simulink model "HVDCMMCInterconnection"  (R2024b)
settings: Solver=FixedStepDiscrete  StartTime=0.0  StopTime=11  RelTol=1e-3
PreLoadFcn:
  | GFLParameters_400Kv
  | HVDCMMCInterconnectionParam
StartFcn:
  | tic
StopFcn:
  | toc
values from neighbouring files (symbols this model uses):
  C_PM = 1.758e-3    (= 0.001758)    [HVDCMMCInterconnectionParam.m]
  Cfilter = 1/(Larm*wc2)    (= 4.78421193241e-05)    [HVDCMMCInterconnectionParam.m]
  Cg = 50e-9    (= 5e-08)    [HVDCMMCInterconnectionParam.m]
  Fc = Fnom*3.37    (= 168.5)    [HVDCMMCInterconnectionParam.m]
  Fnom = 50    [GFLParameters_400Kv.m]    (also in HVDCMMCInterconnectionParam.m)
  L_cable = 15e-3    (= 0.015)    [HVDCMMCInterconnectionParam.m]
  Larm = Larm_pu*(Zbase/(2*pi*Fnom))    (= 0.0529455974536)    [HVDCMMCInterconnectionParam.m]
  Limits_Qreg = [ 0.25, -0.25 ]    [HVDCMMCInterconnectionParam.m]
  Lxfo = 0.12    [HVDCMMCInterconnectionParam.m]
  Nb_PM = 36    [HVDCMMCInterconnectionParam.m]
  Pnom = 1000e6    (= 1000000000)    [HVDCMMCInterconnectionParam.m]
  Psc = Pnom*20    (= 20000000000)    [HVDCMMCInterconnectionParam.m]    (also in HVDCMMC_RunFaultAnalysis.m = gridSCLArray(k))
  R_cable = 0.5    [HVDCMMCInterconnectionParam.m]
  R_startup = 400    [HVDCMMCInterconnectionParam.m]
  Rarm = Rarm_pu*Zbase    (= 0.1663335)    [HVDCMMCInterconnectionParam.m]
  Rfilter = 1/(Cfilter*w)*30    (= 1996.002)    [HVDCMMCInterconnectionParam.m]
  Rg = 100    [HVDCMMCInterconnectionParam.m]
  Rxfo = 0.003    [HVDCMMCInterconnectionParam.m]
  Slope_Pref = 0.5    [HVDCMMCInterconnectionParam.m]
  Slope_Qref = 0.5    [HVDCMMCInterconnectionParam.m]
  Slope_Vdc_ref = Vnom_dc/5    (= 128000)    [HVDCMMCInterconnectionParam.m]
  Tbrk1_On = 0.1    [HVDCMMCInterconnectionParam.m]
  Tbrk2_On = 1.0    (= 1)    [HVDCMMCInterconnectionParam.m]
  Tdeblock = 1.5    [HVDCMMCInterconnectionParam.m]
  Tfault = 9999    [HVDCMMCInterconnectionParam.m]
  Ton_Converter2 = 4    [HVDCMMCInterconnectionParam.m]
  Ton_PQreg = 4    [HVDCMMCInterconnectionParam.m]
  Ton_VDCreg = 1.5    [HVDCMMCInterconnectionParam.m]
  Ts = Ts_Control    (= 4e-05)    [HVDCMMCInterconnectionParam.m]
  Ts_Power = 20e-6    (= 2e-05)    [HVDCMMCInterconnectionParam.m]
  Vnom_dc = 640e3    (= 640000)    [HVDCMMCInterconnectionParam.m]
  Vnom_prim = 400e3    (= 400000)    [HVDCMMCInterconnectionParam.m]
  Vnom_sec = 333e3    (= 333000)    [HVDCMMCInterconnectionParam.m]
undefined symbols (not defined in the file or in its folder): ConvCtrl, ConvPlt, DiscIntNeverNeededParam, Discrete, ee_sli_rtmsupport, Fault, gcbh, gridInverter, magnitude, Pcc, PlantSim, sps, sps_rtmsupport, spsPLL3phModel, TL, Trf
libraries: powerlib_extras x27, spsSeriesRLCBranchLib x27, simulink x14, eeGeneralControl x11, spsCurrentMeasurementLib x11, spsVoltageMeasurementLib x8, spsBreakerLib x7, eeTransforms x6, spsHalfBridgeMMCLib x6, spsSecondOrderFilterLib x4, spsabctodq0Lib x4, spsThreePhaseVIMeasurementLib x4
(part 3 of 6)

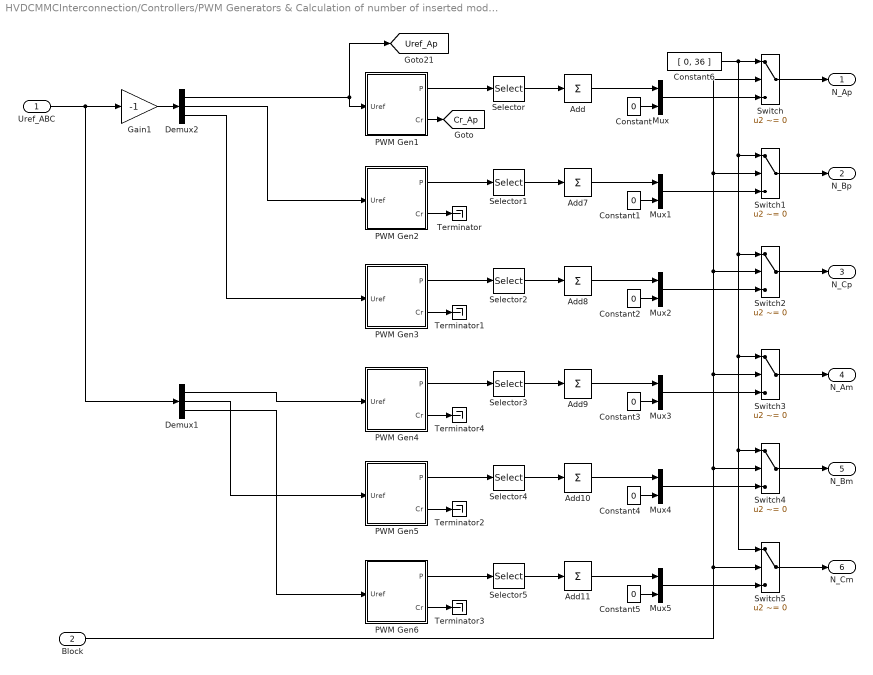
== system HVDCMMCInterconnection/Controllers/PWM Generators & Calculation of number of inserted modules (Nin) and number of blocked module (Nbl) ==
  Uref_ABC : Inport  PortDimensions=3
  Block : Inport  Port=2
  Add{,7..11} (6 alike) : Sum  Inputs=1
  Constant{,1..5} (6 alike) : Constant  Value=0
  Constant6 : Constant  Value=[ 0, 36 ]
  Demux1 : Demux  Outputs=3
  Demux2 : Demux  Outputs=3
  Gain1 : Gain  Gain=-1
  Mux{,1..5} (6 alike) : Mux  Inputs=2
  PWM Gen1 : Subsystem  mask(PWM generator for half-bridge MMC){n=Nb_PM, Fc=Fc, Ts=Ts_Power}
      mask prompts: n "Number of half-bridges"; Fc "Carriers frequency (Hz)"; Ts "Sample time (s)"
      mask init:
      | Tc=1/Fc;
      |         Pc= [ 0:360/n:360-360/n]*pi/180;
      |         Offset=Pc/(2*pi);
      |         Offset_Cr=Pc/(2*pi)*Tc;
      |         p=0;
      |         for m=1:2:2*n
      |             p=p+1;
      |             SelectPulsesPS(m)=p;
      |             SelectPulsesPS(m+1)=p+n;
      |         end
  PWM Gen2 : Subsystem  mask(PWM generator for half-bridge MMC){n=Nb_PM, Fc=Fc, Ts=Ts_Power}
      mask prompts: n "Number of half-bridges"; Fc "Carriers frequency (Hz)"; Ts "Sample time (s)"
      mask init: same as HVDCMMCInterconnection/Controllers/PWM Generators & Calculation of number of inserted modules (Nin) and number of blocked module (Nbl)/PWM Gen1
  PWM Gen3 : Subsystem  mask(PWM generator for half-bridge MMC){n=Nb_PM, Fc=Fc, Ts=Ts_Power}
      mask prompts: n "Number of half-bridges"; Fc "Carriers frequency (Hz)"; Ts "Sample time (s)"
      mask init: same as HVDCMMCInterconnection/Controllers/PWM Generators & Calculation of number of inserted modules (Nin) and number of blocked module (Nbl)/PWM Gen1
  PWM Gen4 : Subsystem  mask(PWM generator for half-bridge MMC){n=Nb_PM, Fc=Fc, Ts=Ts_Power}
      mask prompts: n "Number of half-bridges"; Fc "Carriers frequency (Hz)"; Ts "Sample time (s)"
      mask init: same as HVDCMMCInterconnection/Controllers/PWM Generators & Calculation of number of inserted modules (Nin) and number of blocked module (Nbl)/PWM Gen1
  PWM Gen5 : Subsystem  mask(PWM generator for half-bridge MMC){n=Nb_PM, Fc=Fc, Ts=Ts_Power}
      mask prompts: n "Number of half-bridges"; Fc "Carriers frequency (Hz)"; Ts "Sample time (s)"
      mask init: same as HVDCMMCInterconnection/Controllers/PWM Generators & Calculation of number of inserted modules (Nin) and number of blocked module (Nbl)/PWM Gen1
  PWM Gen6 : Subsystem  mask(PWM generator for half-bridge MMC){n=Nb_PM, Fc=Fc, Ts=Ts_Power}
      mask prompts: n "Number of half-bridges"; Fc "Carriers frequency (Hz)"; Ts "Sample time (s)"
      mask init: same as HVDCMMCInterconnection/Controllers/PWM Generators & Calculation of number of inserted modules (Nin) and number of blocked module (Nbl)/PWM Gen1
  Selector{,1..5} (6 alike) : Selector  InputPortWidth=72  IndexOptions=Index vector (dialog)  Indices=[1:2:71]  OutputSizes=1
  Switch{,1..5} (6 alike) : Switch  Criteria=u2 ~= 0  SaturateOnIntegerOverflow=off  InputSameDT=off
  Terminator{,1..4} (5 alike) : Terminator
  N_Ap : Outport
  N_Bp : Outport  Port=2
  N_Cp : Outport  Port=3
  N_Am : Outport  Port=4
  N_Bm : Outport  Port=5
  N_Cm : Outport  Port=6
  tag scope: Cr_Ap=global, Uref_Ap=global
  wires:
  PWM Gen4/2(Cr) -> Terminator4/1
  PWM Gen5/2(Cr) -> Terminator2/1
  Uref_ABC/1 -> Gain1/1, Demux1/1
  PWM Gen6/2(Cr) -> Terminator3/1
  PWM Gen2/2(Cr) -> Terminator/1
  Demux2/2 -> PWM Gen2/1(Uref)
  Demux2/1 -> PWM Gen1/1(Uref), [Uref_Ap]
  Gain1/1 -> Demux2/1
  PWM Gen1/2(Cr) -> [Cr_Ap]
  PWM Gen3/2(Cr) -> Terminator1/1
  Selector/1 -> Add/1
  Selector1/1 -> Add7/1
  Selector2/1 -> Add8/1
  Selector3/1 -> Add9/1
  Selector4/1 -> Add10/1
  Selector5/1 -> Add11/1
  Constant/1 -> Mux/2
  Add7/1 -> Mux1/1
  Constant1/1 -> Mux1/2
  Constant5/1 -> Mux5/2
  Switch/1 -> N_Ap/1
  Switch3/1 -> N_Am/1
  Mux1/1 -> Switch1/3
  Constant6/1 -> Switch/1, Switch5/1, Switch4/1, Switch3/1, Switch2/1, Switch1/1
  Constant2/1 -> Mux2/2
  Add9/1 -> Mux3/1
  Add8/1 -> Mux2/1
  Mux/1 -> Switch/3
  Switch1/1 -> N_Bp/1
  Constant4/1 -> Mux4/2
  Switch2/1 -> N_Cp/1
  Switch4/1 -> N_Bm/1
  Add/1 -> Mux/1
  Switch5/1 -> N_Cm/1
  Constant3/1 -> Mux3/2
  Add10/1 -> Mux4/1
  Add11/1 -> Mux5/1
  Block/1 -> Switch/2, Switch1/2, Switch2/2, Switch3/2, Switch4/2, Switch5/2
  Mux3/1 -> Switch3/3
  Mux4/1 -> Switch4/3
  Mux5/1 -> Switch5/3
  Mux2/1 -> Switch2/3
  PWM Gen6/1(P) -> Selector5/1
  PWM Gen5/1(P) -> Selector4/1
  PWM Gen4/1(P) -> Selector3/1
  PWM Gen3/1(P) -> Selector2/1
  PWM Gen2/1(P) -> Selector1/1
  PWM Gen1/1(P) -> Selector/1
  Demux2/3 -> PWM Gen3/1(Uref)
  Demux1/1 -> PWM Gen4/1(Uref)
  Demux1/3 -> PWM Gen6/1(Uref)
  Demux1/2 -> PWM Gen5/1(Uref)

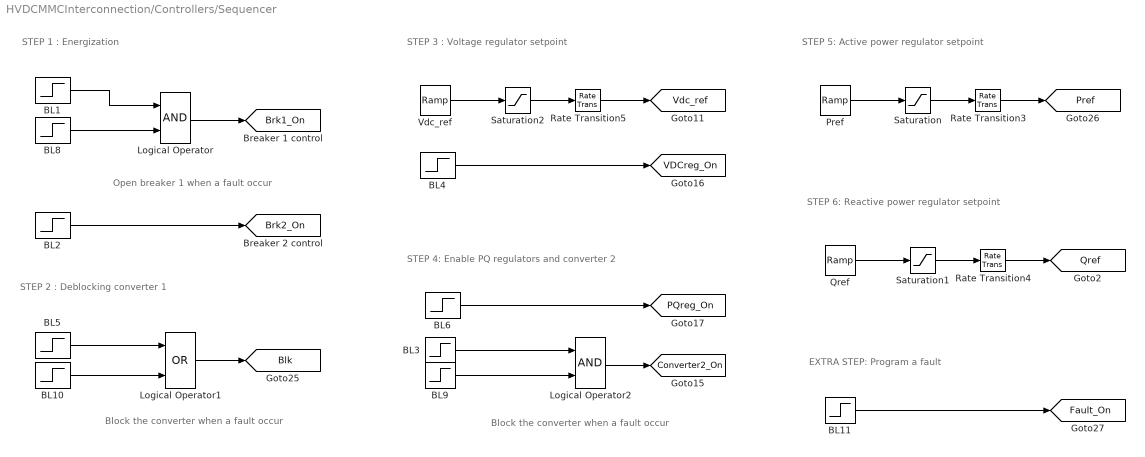
== system HVDCMMCInterconnection/Controllers/Sequencer ==
  note: Open breaker 1 when a fault occur
  note: Block the converter when a fault occur
  note: Block the converter when a fault occur
  note: STEP 6: Reactive power regulator setpoint
  note: STEP 4: Enable PQ regulators and converter 2
  note: STEP 5: Active power regulator setpoint
  note: STEP 3 : Voltage regulator setpoint
  note: STEP 2 : Deblocking converter 1
  note: STEP 1 : Energization
  note: EXTRA STEP: Program a fault
  BL1 : Step  Time=Tbrk1_On  SampleTime=Ts_Power
  BL10 : Step  Time=Tfault+Ts_Power  SampleTime=Ts_Power
  BL11 : Step  Time=Tfault  SampleTime=Ts_Power
  BL2 : Step  Time=Tbrk2_On  SampleTime=Ts_Power
  BL3 : Step  Time=Ton_Converter2  SampleTime=Ts_Power
  BL4 : Step  Time=Ton_VDCreg  SampleTime=Ts
  BL5 : Step  Time=Tdeblock  Before=1  After=0  SampleTime=Ts_Power
  BL6 : Step  Time=Ton_PQreg  SampleTime=Ts
  BL8 : Step  Time=Tfault + 1.95*(1/Fnom)  Before=1  After=0  SampleTime=Ts_Power
  BL9 : Step  Time=Tfault + 2*(1/Fnom)  Before=1  After=0  SampleTime=Ts_Power
  Logical Operator : Logic  AllPortsSameDT=off  OutDataTypeStr=boolean
  Logical Operator1 : Logic  Operator=OR  AllPortsSameDT=off  OutDataTypeStr=float('double')
  Logical Operator2 : Logic  AllPortsSameDT=off  OutDataTypeStr=boolean
  Pref : simulink/Sources/Ramp  slope=Slope_Pref  start=Tramping_Pref  InitialOutput=0
  Qref : simulink/Sources/Ramp  slope=Slope_Qref  start=Tramping_Qref  InitialOutput=0
  Rate Transition3 : RateTransition  OutPortSampleTime=Ts_Control
  Rate Transition4 : RateTransition  OutPortSampleTime=Ts_Control
  Rate Transition5 : RateTransition  OutPortSampleTime=Ts_Control
  Saturation : Saturate  UpperLimit=1  LowerLimit=-1
  Saturation1 : Saturate  UpperLimit=Limits_Qreg(1)  LowerLimit=Limits_Qreg(2)
  Saturation2 : Saturate  UpperLimit=Vnom_dc  LowerLimit=eps
  "Vdc_ref " : simulink/Sources/Ramp  slope=Slope_Vdc_ref  start=Tramping_Vdc_ref  InitialOutput=Vnom_sec*1.37
  tag scope: Blk=global, Brk1_On=global, Brk2_On=global, Converter2_On=global, Fault_On=global, PQreg_On=global, Pref=global, Qref=global, VDCreg_On=global, Vdc_ref=global
  wires:
  Saturation2/1 -> Rate Transition5/1
  Saturation1/1 -> Rate Transition4/1
  Pref/1 -> Saturation/1
  Qref/1 -> Saturation1/1
  Saturation/1 -> Rate Transition3/1
  Rate Transition3/1 -> [Pref]
  Rate Transition4/1 -> [Qref]
  Rate Transition5/1 -> [Vdc_ref]
  BL4/1 -> [VDCreg_On]
  BL6/1 -> [PQreg_On]
  "Vdc_ref "/1 -> Saturation2/1
  BL2/1 -> [Brk2_On]
  BL8/1 -> Logical Operator/2
  Logical Operator/1 -> [Brk1_On]
  BL1/1 -> Logical Operator/1
  BL9/1 -> Logical Operator2/2
  BL3/1 -> Logical Operator2/1
  Logical Operator2/1 -> [Converter2_On]
  Logical Operator1/1 -> [Blk]
  BL5/1 -> Logical Operator1/1
  BL10/1 -> Logical Operator1/2
  BL11/1 -> [Fault_On]

== system HVDCMMCInterconnection/Record Simulation Data/FaultTrigger ==
  mZ1L_Est : Inport
  V1_Local : Inport  Port=2
  I1_Local : Inport  Port=3
  V1_Remote : Inport  Port=4
  I1_Remote : Inport  Port=5
  IdRef : Inport  Port=6
  IqRef : Inport  Port=7
  IdMeas : Inport  Port=8
  IqMeas : Inport  Port=9
  Is : Inport  Port=10
  Vmd : Inport  Port=11
  Vmq : Inport  Port=12
  delVd : Inport  Port=13
  delVq : Inport  Port=14
  Enable : EnablePort
  To Workspace : ToWorkspace  VariableName=mZ1L_Est  SaveFormat=Timeseries  SampleTime=-1
  To Workspace1 : ToWorkspace  VariableName=V1_Local  SaveFormat=Timeseries  SampleTime=-1
  To Workspace10 : ToWorkspace  VariableName=Vmd  SaveFormat=Timeseries  SampleTime=-1
  To Workspace11 : ToWorkspace  VariableName=Vmq  SaveFormat=Timeseries  SampleTime=-1
  To Workspace12 : ToWorkspace  VariableName=delVd  SaveFormat=Timeseries  SampleTime=-1
  To Workspace13 : ToWorkspace  VariableName=delVq  SaveFormat=Timeseries  SampleTime=-1
  To Workspace2 : ToWorkspace  VariableName=I1_Local  SaveFormat=Timeseries  SampleTime=-1
  To Workspace3 : ToWorkspace  VariableName=V1_Remote  SaveFormat=Timeseries  SampleTime=-1
  To Workspace4 : ToWorkspace  VariableName=I1_Remote  SaveFormat=Timeseries  SampleTime=-1
  To Workspace5 : ToWorkspace  VariableName=IdRef  SaveFormat=Timeseries  SampleTime=-1
  To Workspace6 : ToWorkspace  VariableName=IqRef  SaveFormat=Timeseries  SampleTime=-1
  To Workspace7 : ToWorkspace  VariableName=IdMeas  SaveFormat=Timeseries  SampleTime=-1
  To Workspace8 : ToWorkspace  VariableName=IqMeas  SaveFormat=Timeseries  SampleTime=-1
  To Workspace9 : ToWorkspace  VariableName=Is  SaveFormat=Timeseries  SampleTime=-1
  wires:
  mZ1L_Est/1 -> To Workspace/1
  V1_Local/1 -> To Workspace1/1
  I1_Local/1 -> To Workspace2/1
  V1_Remote/1 -> To Workspace3/1
  I1_Remote/1 -> To Workspace4/1
  IdRef/1 -> To Workspace5/1
  IqRef/1 -> To Workspace6/1
  IdMeas/1 -> To Workspace7/1
  IqMeas/1 -> To Workspace8/1
  Is/1 -> To Workspace9/1
  Vmd/1 -> To Workspace10/1
  Vmq/1 -> To Workspace11/1
  delVd/1 -> To Workspace12/1
  delVq/1 -> To Workspace13/1

== system HVDCMMCInterconnection/BusCalculations/Measurement Unit (Phasor Computation)/Discrete Fourier(A) ==
  note: Discrete Fourier
  note: Pierre Giroux, Gilbert Sybille
      | Power System Simulation Laboratory
      | IREQ, Hydro-Quebc
  In : Inport
  Demux : Demux  Outputs=2
      settings: DisplayOption=none
  Discrete Mean value1 : powerlib_extras/Discrete Measurements/Discrete  Mean value  Freq=Freq  Vinit=Real_Init  Ts=Ts
  Discrete Mean value2 : powerlib_extras/Discrete Measurements/Discrete  Mean value  Freq=Freq  Vinit=Imag_Init  Ts=Ts
  Gain : Gain  Gain=2*pi*n*Freq  SaturateOnIntegerOverflow=on  OutDataTypeStr=Inherit: Same as input  ParamDataTypeStr=Inherit: Same as input
  Gain1 : Gain  Gain=k  SaturateOnIntegerOverflow=on  OutDataTypeStr=Inherit: Same as input  ParamDataTypeStr=Inherit: Same as input
  Mux : Mux  Inputs=2
  Product : Product  InputSameDT=on  SaturateOnIntegerOverflow=on  OutDataTypeStr=Inherit: Same as first input
  Real-Imag to Complex : RealImagToComplex
  Trigonometric Function : Trigonometry
  Trigonometric Function1 : Trigonometry  Operator=cos
  t : DigitalClock  SampleTime=Ts
  Fund : Outport
  wires:
  Real-Imag to Complex/1 -> Fund/1
  Discrete Mean value2/1 -> Real-Imag to Complex/2  "Imag"
  Discrete Mean value1/1 -> Real-Imag to Complex/1  "Real"
  t/1 -> Gain/1
  Gain/1 -> Trigonometric Function/1, Trigonometric Function1/1
  Trigonometric Function/1 -> Mux/1
  Trigonometric Function1/1 -> Mux/2
  Mux/1 -> Gain1/1
  In/1 -> Product/1
  Gain1/1 -> Product/2
  Product/1 -> Demux/1
  Demux/1 -> Discrete Mean value1/1
  Demux/2 -> Discrete Mean value2/1

== system HVDCMMCInterconnection/BusCalculations/Measurement Unit (Phasor Computation)/Discrete Fourier(A)  ==
  note: Pierre Giroux, Gilbert Sybille
      | Power System Simulation Laboratory
      | IREQ, Hydro-Quebc
  note: Discrete Fourier
  In : Inport
  Demux : Demux  Outputs=2
      settings: DisplayOption=none
  Discrete Mean value1 : powerlib_extras/Discrete Measurements/Discrete  Mean value  Freq=Freq  Vinit=Real_Init  Ts=Ts
  Discrete Mean value2 : powerlib_extras/Discrete Measurements/Discrete  Mean value  Freq=Freq  Vinit=Imag_Init  Ts=Ts
  Gain : Gain  Gain=2*pi*n*Freq  SaturateOnIntegerOverflow=on  OutDataTypeStr=Inherit: Same as input  ParamDataTypeStr=Inherit: Same as input
  Gain1 : Gain  Gain=k  SaturateOnIntegerOverflow=on  OutDataTypeStr=Inherit: Same as input  ParamDataTypeStr=Inherit: Same as input
  Mux : Mux  Inputs=2
  Product : Product  InputSameDT=on  SaturateOnIntegerOverflow=on  OutDataTypeStr=Inherit: Same as first input
  Real-Imag to Complex : RealImagToComplex
  Trigonometric Function : Trigonometry
  Trigonometric Function1 : Trigonometry  Operator=cos
  t : DigitalClock  SampleTime=Ts
  Fund : Outport
  wires:
  Demux/2 -> Discrete Mean value2/1
  Demux/1 -> Discrete Mean value1/1
  Product/1 -> Demux/1
  Gain1/1 -> Product/2
  In/1 -> Product/1
  Mux/1 -> Gain1/1
  Trigonometric Function1/1 -> Mux/2
  Trigonometric Function/1 -> Mux/1
  Gain/1 -> Trigonometric Function1/1, Trigonometric Function/1
  t/1 -> Gain/1
  Discrete Mean value1/1 -> Real-Imag to Complex/1  "Real"
  Discrete Mean value2/1 -> Real-Imag to Complex/2  "Imag"
  Real-Imag to Complex/1 -> Fund/1

== system HVDCMMCInterconnection/BusCalculations/Measurement Unit (Phasor Computation)/Discrete Fourier(B) ==
  note: Pierre Giroux, Gilbert Sybille
      | Power System Simulation Laboratory
      | IREQ, Hydro-Quebc
  note: Discrete Fourier
  In : Inport
  Demux : Demux  Outputs=2
      settings: DisplayOption=none
  Discrete Mean value1 : powerlib_extras/Discrete Measurements/Discrete  Mean value  Freq=Freq  Vinit=Real_Init  Ts=Ts
  Discrete Mean value2 : powerlib_extras/Discrete Measurements/Discrete  Mean value  Freq=Freq  Vinit=Imag_Init  Ts=Ts
  Gain : Gain  Gain=2*pi*n*Freq  SaturateOnIntegerOverflow=on  OutDataTypeStr=Inherit: Same as input  ParamDataTypeStr=Inherit: Same as input
  Gain1 : Gain  Gain=k  SaturateOnIntegerOverflow=on  OutDataTypeStr=Inherit: Same as input  ParamDataTypeStr=Inherit: Same as input
  Mux : Mux  Inputs=2
  Product : Product  InputSameDT=on  SaturateOnIntegerOverflow=on  OutDataTypeStr=Inherit: Same as first input
  Real-Imag to Complex : RealImagToComplex
  Trigonometric Function : Trigonometry
  Trigonometric Function1 : Trigonometry  Operator=cos
  t : DigitalClock  SampleTime=Ts
  Fund : Outport
  wires:
  Demux/2 -> Discrete Mean value2/1
  Demux/1 -> Discrete Mean value1/1
  Product/1 -> Demux/1
  Gain1/1 -> Product/2
  In/1 -> Product/1
  Mux/1 -> Gain1/1
  Trigonometric Function1/1 -> Mux/2
  Trigonometric Function/1 -> Mux/1
  Gain/1 -> Trigonometric Function1/1, Trigonometric Function/1
  t/1 -> Gain/1
  Discrete Mean value1/1 -> Real-Imag to Complex/1  "Real"
  Discrete Mean value2/1 -> Real-Imag to Complex/2  "Imag"
  Real-Imag to Complex/1 -> Fund/1

== system HVDCMMCInterconnection/BusCalculations/Measurement Unit (Phasor Computation)/Discrete Fourier(B)  ==
  note: Discrete Fourier
  note: Pierre Giroux, Gilbert Sybille
      | Power System Simulation Laboratory
      | IREQ, Hydro-Quebc
  In : Inport
  Demux : Demux  Outputs=2
      settings: DisplayOption=none
  Discrete Mean value1 : powerlib_extras/Discrete Measurements/Discrete  Mean value  Freq=Freq  Vinit=Real_Init  Ts=Ts
  Discrete Mean value2 : powerlib_extras/Discrete Measurements/Discrete  Mean value  Freq=Freq  Vinit=Imag_Init  Ts=Ts
  Gain : Gain  Gain=2*pi*n*Freq  SaturateOnIntegerOverflow=on  OutDataTypeStr=Inherit: Same as input  ParamDataTypeStr=Inherit: Same as input
  Gain1 : Gain  Gain=k  SaturateOnIntegerOverflow=on  OutDataTypeStr=Inherit: Same as input  ParamDataTypeStr=Inherit: Same as input
  Mux : Mux  Inputs=2
  Product : Product  InputSameDT=on  SaturateOnIntegerOverflow=on  OutDataTypeStr=Inherit: Same as first input
  Real-Imag to Complex : RealImagToComplex
  Trigonometric Function : Trigonometry
  Trigonometric Function1 : Trigonometry  Operator=cos
  t : DigitalClock  SampleTime=Ts
  Fund : Outport
  wires:
  Real-Imag to Complex/1 -> Fund/1
  Discrete Mean value2/1 -> Real-Imag to Complex/2  "Imag"
  Discrete Mean value1/1 -> Real-Imag to Complex/1  "Real"
  t/1 -> Gain/1
  Gain/1 -> Trigonometric Function/1, Trigonometric Function1/1
  Trigonometric Function/1 -> Mux/1
  Trigonometric Function1/1 -> Mux/2
  Mux/1 -> Gain1/1
  In/1 -> Product/1
  Gain1/1 -> Product/2
  Product/1 -> Demux/1
  Demux/1 -> Discrete Mean value1/1
  Demux/2 -> Discrete Mean value2/1

== system HVDCMMCInterconnection/BusCalculations/Measurement Unit (Phasor Computation)/Discrete Fourier(C) ==
  note: Discrete Fourier
  note: Pierre Giroux, Gilbert Sybille
      | Power System Simulation Laboratory
      | IREQ, Hydro-Quebc
  In : Inport
  Demux : Demux  Outputs=2
      settings: DisplayOption=none
  Discrete Mean value1 : powerlib_extras/Discrete Measurements/Discrete  Mean value  Freq=Freq  Vinit=Real_Init  Ts=Ts
  Discrete Mean value2 : powerlib_extras/Discrete Measurements/Discrete  Mean value  Freq=Freq  Vinit=Imag_Init  Ts=Ts
  Gain : Gain  Gain=2*pi*n*Freq  SaturateOnIntegerOverflow=on  OutDataTypeStr=Inherit: Same as input  ParamDataTypeStr=Inherit: Same as input
  Gain1 : Gain  Gain=k  SaturateOnIntegerOverflow=on  OutDataTypeStr=Inherit: Same as input  ParamDataTypeStr=Inherit: Same as input
  Mux : Mux  Inputs=2
  Product : Product  InputSameDT=on  SaturateOnIntegerOverflow=on  OutDataTypeStr=Inherit: Same as first input
  Real-Imag to Complex : RealImagToComplex
  Trigonometric Function : Trigonometry
  Trigonometric Function1 : Trigonometry  Operator=cos
  t : DigitalClock  SampleTime=Ts
  Fund : Outport
  wires:
  Real-Imag to Complex/1 -> Fund/1
  Discrete Mean value2/1 -> Real-Imag to Complex/2  "Imag"
  Discrete Mean value1/1 -> Real-Imag to Complex/1  "Real"
  t/1 -> Gain/1
  Gain/1 -> Trigonometric Function/1, Trigonometric Function1/1
  Trigonometric Function/1 -> Mux/1
  Trigonometric Function1/1 -> Mux/2
  Mux/1 -> Gain1/1
  In/1 -> Product/1
  Gain1/1 -> Product/2
  Product/1 -> Demux/1
  Demux/1 -> Discrete Mean value1/1
  Demux/2 -> Discrete Mean value2/1

== system HVDCMMCInterconnection/BusCalculations/Measurement Unit (Phasor Computation)/Discrete Fourier(C)  ==
  note: Pierre Giroux, Gilbert Sybille
      | Power System Simulation Laboratory
      | IREQ, Hydro-Quebc
  note: Discrete Fourier
  In : Inport
  Demux : Demux  Outputs=2
      settings: DisplayOption=none
  Discrete Mean value1 : powerlib_extras/Discrete Measurements/Discrete  Mean value  Freq=Freq  Vinit=Real_Init  Ts=Ts
  Discrete Mean value2 : powerlib_extras/Discrete Measurements/Discrete  Mean value  Freq=Freq  Vinit=Imag_Init  Ts=Ts
  Gain : Gain  Gain=2*pi*n*Freq  SaturateOnIntegerOverflow=on  OutDataTypeStr=Inherit: Same as input  ParamDataTypeStr=Inherit: Same as input
  Gain1 : Gain  Gain=k  SaturateOnIntegerOverflow=on  OutDataTypeStr=Inherit: Same as input  ParamDataTypeStr=Inherit: Same as input
  Mux : Mux  Inputs=2
  Product : Product  InputSameDT=on  SaturateOnIntegerOverflow=on  OutDataTypeStr=Inherit: Same as first input
  Real-Imag to Complex : RealImagToComplex
  Trigonometric Function : Trigonometry
  Trigonometric Function1 : Trigonometry  Operator=cos
  t : DigitalClock  SampleTime=Ts
  Fund : Outport
  wires:
  Demux/2 -> Discrete Mean value2/1
  Demux/1 -> Discrete Mean value1/1
  Product/1 -> Demux/1
  Gain1/1 -> Product/2
  In/1 -> Product/1
  Mux/1 -> Gain1/1
  Trigonometric Function1/1 -> Mux/2
  Trigonometric Function/1 -> Mux/1
  Gain/1 -> Trigonometric Function1/1, Trigonometric Function/1
  t/1 -> Gain/1
  Discrete Mean value1/1 -> Real-Imag to Complex/1  "Real"
  Discrete Mean value2/1 -> Real-Imag to Complex/2  "Imag"
  Real-Imag to Complex/1 -> Fund/1

== system HVDCMMCInterconnection/BusCalculations1/Measurement Unit (Phasor Computation)/Discrete Fourier(A) ==
  note: Pierre Giroux, Gilbert Sybille
      | Power System Simulation Laboratory
      | IREQ, Hydro-Quebc
  note: Discrete Fourier
  In : Inport
  Demux : Demux  Outputs=2
      settings: DisplayOption=none
  Discrete Mean value1 : powerlib_extras/Discrete Measurements/Discrete  Mean value  Freq=Freq  Vinit=Real_Init  Ts=Ts
  Discrete Mean value2 : powerlib_extras/Discrete Measurements/Discrete  Mean value  Freq=Freq  Vinit=Imag_Init  Ts=Ts
  Gain : Gain  Gain=2*pi*n*Freq  SaturateOnIntegerOverflow=on  OutDataTypeStr=Inherit: Same as input  ParamDataTypeStr=Inherit: Same as input
  Gain1 : Gain  Gain=k  SaturateOnIntegerOverflow=on  OutDataTypeStr=Inherit: Same as input  ParamDataTypeStr=Inherit: Same as input
  Mux : Mux  Inputs=2
  Product : Product  InputSameDT=on  SaturateOnIntegerOverflow=on  OutDataTypeStr=Inherit: Same as first input
  Real-Imag to Complex : RealImagToComplex
  Trigonometric Function : Trigonometry
  Trigonometric Function1 : Trigonometry  Operator=cos
  t : DigitalClock  SampleTime=Ts
  Fund : Outport
  wires:
  Demux/2 -> Discrete Mean value2/1
  Demux/1 -> Discrete Mean value1/1
  Product/1 -> Demux/1
  Gain1/1 -> Product/2
  In/1 -> Product/1
  Mux/1 -> Gain1/1
  Trigonometric Function1/1 -> Mux/2
  Trigonometric Function/1 -> Mux/1
  Gain/1 -> Trigonometric Function1/1, Trigonometric Function/1
  t/1 -> Gain/1
  Discrete Mean value1/1 -> Real-Imag to Complex/1  "Real"
  Discrete Mean value2/1 -> Real-Imag to Complex/2  "Imag"
  Real-Imag to Complex/1 -> Fund/1

== system HVDCMMCInterconnection/BusCalculations1/Measurement Unit (Phasor Computation)/Discrete Fourier(A)  ==
  note: Discrete Fourier
  note: Pierre Giroux, Gilbert Sybille
      | Power System Simulation Laboratory
      | IREQ, Hydro-Quebc
  In : Inport
  Demux : Demux  Outputs=2
      settings: DisplayOption=none
  Discrete Mean value1 : powerlib_extras/Discrete Measurements/Discrete  Mean value  Freq=Freq  Vinit=Real_Init  Ts=Ts
  Discrete Mean value2 : powerlib_extras/Discrete Measurements/Discrete  Mean value  Freq=Freq  Vinit=Imag_Init  Ts=Ts
  Gain : Gain  Gain=2*pi*n*Freq  SaturateOnIntegerOverflow=on  OutDataTypeStr=Inherit: Same as input  ParamDataTypeStr=Inherit: Same as input
  Gain1 : Gain  Gain=k  SaturateOnIntegerOverflow=on  OutDataTypeStr=Inherit: Same as input  ParamDataTypeStr=Inherit: Same as input
  Mux : Mux  Inputs=2
  Product : Product  InputSameDT=on  SaturateOnIntegerOverflow=on  OutDataTypeStr=Inherit: Same as first input
  Real-Imag to Complex : RealImagToComplex
  Trigonometric Function : Trigonometry
  Trigonometric Function1 : Trigonometry  Operator=cos
  t : DigitalClock  SampleTime=Ts
  Fund : Outport
  wires:
  Real-Imag to Complex/1 -> Fund/1
  Discrete Mean value2/1 -> Real-Imag to Complex/2  "Imag"
  Discrete Mean value1/1 -> Real-Imag to Complex/1  "Real"
  t/1 -> Gain/1
  Gain/1 -> Trigonometric Function/1, Trigonometric Function1/1
  Trigonometric Function/1 -> Mux/1
  Trigonometric Function1/1 -> Mux/2
  Mux/1 -> Gain1/1
  In/1 -> Product/1
  Gain1/1 -> Product/2
  Product/1 -> Demux/1
  Demux/1 -> Discrete Mean value1/1
  Demux/2 -> Discrete Mean value2/1

== system HVDCMMCInterconnection/BusCalculations1/Measurement Unit (Phasor Computation)/Discrete Fourier(B) ==
  note: Discrete Fourier
  note: Pierre Giroux, Gilbert Sybille
      | Power System Simulation Laboratory
      | IREQ, Hydro-Quebc
  In : Inport
  Demux : Demux  Outputs=2
      settings: DisplayOption=none
  Discrete Mean value1 : powerlib_extras/Discrete Measurements/Discrete  Mean value  Freq=Freq  Vinit=Real_Init  Ts=Ts
  Discrete Mean value2 : powerlib_extras/Discrete Measurements/Discrete  Mean value  Freq=Freq  Vinit=Imag_Init  Ts=Ts
  Gain : Gain  Gain=2*pi*n*Freq  SaturateOnIntegerOverflow=on  OutDataTypeStr=Inherit: Same as input  ParamDataTypeStr=Inherit: Same as input
  Gain1 : Gain  Gain=k  SaturateOnIntegerOverflow=on  OutDataTypeStr=Inherit: Same as input  ParamDataTypeStr=Inherit: Same as input
  Mux : Mux  Inputs=2
  Product : Product  InputSameDT=on  SaturateOnIntegerOverflow=on  OutDataTypeStr=Inherit: Same as first input
  Real-Imag to Complex : RealImagToComplex
  Trigonometric Function : Trigonometry
  Trigonometric Function1 : Trigonometry  Operator=cos
  t : DigitalClock  SampleTime=Ts
  Fund : Outport
  wires:
  Real-Imag to Complex/1 -> Fund/1
  Discrete Mean value2/1 -> Real-Imag to Complex/2  "Imag"
  Discrete Mean value1/1 -> Real-Imag to Complex/1  "Real"
  t/1 -> Gain/1
  Gain/1 -> Trigonometric Function/1, Trigonometric Function1/1
  Trigonometric Function/1 -> Mux/1
  Trigonometric Function1/1 -> Mux/2
  Mux/1 -> Gain1/1
  In/1 -> Product/1
  Gain1/1 -> Product/2
  Product/1 -> Demux/1
  Demux/1 -> Discrete Mean value1/1
  Demux/2 -> Discrete Mean value2/1

== system HVDCMMCInterconnection/BusCalculations1/Measurement Unit (Phasor Computation)/Discrete Fourier(B)  ==
  note: Pierre Giroux, Gilbert Sybille
      | Power System Simulation Laboratory
      | IREQ, Hydro-Quebc
  note: Discrete Fourier
  In : Inport
  Demux : Demux  Outputs=2
      settings: DisplayOption=none
  Discrete Mean value1 : powerlib_extras/Discrete Measurements/Discrete  Mean value  Freq=Freq  Vinit=Real_Init  Ts=Ts
  Discrete Mean value2 : powerlib_extras/Discrete Measurements/Discrete  Mean value  Freq=Freq  Vinit=Imag_Init  Ts=Ts
  Gain : Gain  Gain=2*pi*n*Freq  SaturateOnIntegerOverflow=on  OutDataTypeStr=Inherit: Same as input  ParamDataTypeStr=Inherit: Same as input
  Gain1 : Gain  Gain=k  SaturateOnIntegerOverflow=on  OutDataTypeStr=Inherit: Same as input  ParamDataTypeStr=Inherit: Same as input
  Mux : Mux  Inputs=2
  Product : Product  InputSameDT=on  SaturateOnIntegerOverflow=on  OutDataTypeStr=Inherit: Same as first input
  Real-Imag to Complex : RealImagToComplex
  Trigonometric Function : Trigonometry
  Trigonometric Function1 : Trigonometry  Operator=cos
  t : DigitalClock  SampleTime=Ts
  Fund : Outport
  wires:
  Demux/2 -> Discrete Mean value2/1
  Demux/1 -> Discrete Mean value1/1
  Product/1 -> Demux/1
  Gain1/1 -> Product/2
  In/1 -> Product/1
  Mux/1 -> Gain1/1
  Trigonometric Function1/1 -> Mux/2
  Trigonometric Function/1 -> Mux/1
  Gain/1 -> Trigonometric Function1/1, Trigonometric Function/1
  t/1 -> Gain/1
  Discrete Mean value1/1 -> Real-Imag to Complex/1  "Real"
  Discrete Mean value2/1 -> Real-Imag to Complex/2  "Imag"
  Real-Imag to Complex/1 -> Fund/1

== system HVDCMMCInterconnection/BusCalculations1/Measurement Unit (Phasor Computation)/Discrete Fourier(C) ==
  note: Pierre Giroux, Gilbert Sybille
      | Power System Simulation Laboratory
      | IREQ, Hydro-Quebc
  note: Discrete Fourier
  In : Inport
  Demux : Demux  Outputs=2
      settings: DisplayOption=none
  Discrete Mean value1 : powerlib_extras/Discrete Measurements/Discrete  Mean value  Freq=Freq  Vinit=Real_Init  Ts=Ts
  Discrete Mean value2 : powerlib_extras/Discrete Measurements/Discrete  Mean value  Freq=Freq  Vinit=Imag_Init  Ts=Ts
  Gain : Gain  Gain=2*pi*n*Freq  SaturateOnIntegerOverflow=on  OutDataTypeStr=Inherit: Same as input  ParamDataTypeStr=Inherit: Same as input
  Gain1 : Gain  Gain=k  SaturateOnIntegerOverflow=on  OutDataTypeStr=Inherit: Same as input  ParamDataTypeStr=Inherit: Same as input
  Mux : Mux  Inputs=2
  Product : Product  InputSameDT=on  SaturateOnIntegerOverflow=on  OutDataTypeStr=Inherit: Same as first input
  Real-Imag to Complex : RealImagToComplex
  Trigonometric Function : Trigonometry
  Trigonometric Function1 : Trigonometry  Operator=cos
  t : DigitalClock  SampleTime=Ts
  Fund : Outport
  wires:
  Demux/2 -> Discrete Mean value2/1
  Demux/1 -> Discrete Mean value1/1
  Product/1 -> Demux/1
  Gain1/1 -> Product/2
  In/1 -> Product/1
  Mux/1 -> Gain1/1
  Trigonometric Function1/1 -> Mux/2
  Trigonometric Function/1 -> Mux/1
  Gain/1 -> Trigonometric Function1/1, Trigonometric Function/1
  t/1 -> Gain/1
  Discrete Mean value1/1 -> Real-Imag to Complex/1  "Real"
  Discrete Mean value2/1 -> Real-Imag to Complex/2  "Imag"
  Real-Imag to Complex/1 -> Fund/1

== system HVDCMMCInterconnection/BusCalculations1/Measurement Unit (Phasor Computation)/Discrete Fourier(C)  ==
  note: Discrete Fourier
  note: Pierre Giroux, Gilbert Sybille
      | Power System Simulation Laboratory
      | IREQ, Hydro-Quebc
  In : Inport
  Demux : Demux  Outputs=2
      settings: DisplayOption=none
  Discrete Mean value1 : powerlib_extras/Discrete Measurements/Discrete  Mean value  Freq=Freq  Vinit=Real_Init  Ts=Ts
  Discrete Mean value2 : powerlib_extras/Discrete Measurements/Discrete  Mean value  Freq=Freq  Vinit=Imag_Init  Ts=Ts
  Gain : Gain  Gain=2*pi*n*Freq  SaturateOnIntegerOverflow=on  OutDataTypeStr=Inherit: Same as input  ParamDataTypeStr=Inherit: Same as input
  Gain1 : Gain  Gain=k  SaturateOnIntegerOverflow=on  OutDataTypeStr=Inherit: Same as input  ParamDataTypeStr=Inherit: Same as input
  Mux : Mux  Inputs=2
  Product : Product  InputSameDT=on  SaturateOnIntegerOverflow=on  OutDataTypeStr=Inherit: Same as first input
  Real-Imag to Complex : RealImagToComplex
  Trigonometric Function : Trigonometry
  Trigonometric Function1 : Trigonometry  Operator=cos
  t : DigitalClock  SampleTime=Ts
  Fund : Outport
  wires:
  Real-Imag to Complex/1 -> Fund/1
  Discrete Mean value2/1 -> Real-Imag to Complex/2  "Imag"
  Discrete Mean value1/1 -> Real-Imag to Complex/1  "Real"
  t/1 -> Gain/1
  Gain/1 -> Trigonometric Function/1, Trigonometric Function1/1
  Trigonometric Function/1 -> Mux/1
  Trigonometric Function1/1 -> Mux/2
  Mux/1 -> Gain1/1
  In/1 -> Product/1
  Gain1/1 -> Product/2
  Product/1 -> Demux/1
  Demux/1 -> Discrete Mean value1/1
  Demux/2 -> Discrete Mean value2/1

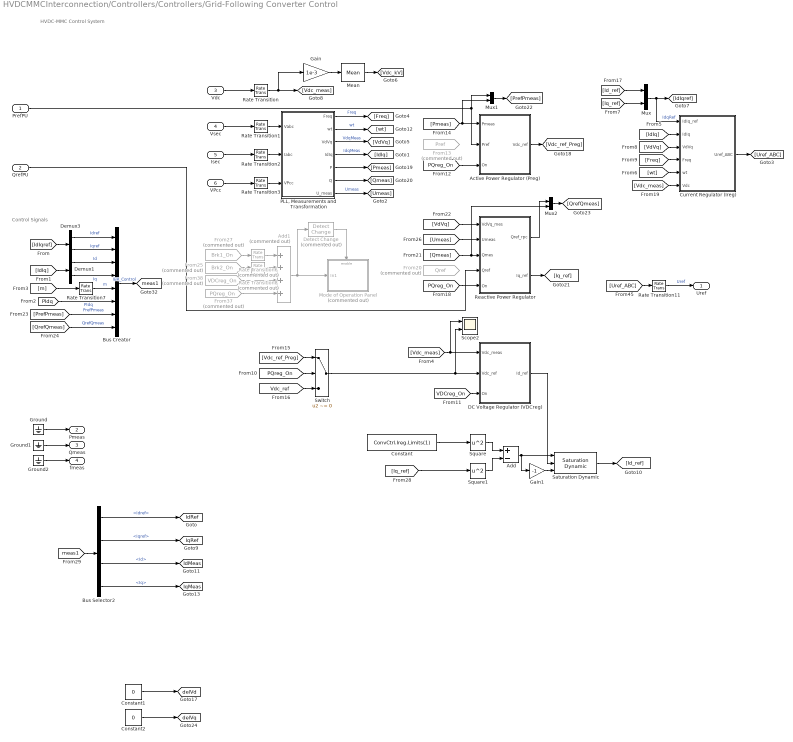
== system HVDCMMCInterconnection/Controllers/Controllers/Grid-Following Converter Control ==
  note: Control Signals
  note: HVDC-MMC Control System
  PrefPU : Inport
  QrefPU : Inport  Port=2
  Vdc : Inport  Port=3
  Vsec : Inport  Port=4
  Isec : Inport  Port=5
  VPcc : Inport  Port=6
  Active Power Regulator (Preg) : Subsystem
  Add : Sum  Inputs=+-
  Add1 : Sum  Commented=on  Inputs=++++
  Bus Creator : BusCreator  Inputs=8
  Bus Selector2 : BusSelector  OutputSignals=Idref,Iqref,Id,Iq
  Constant : Constant  Value=ConvCtrl.Ireg.Limits(1)
  Constant1 : Constant  Value=0
  Constant2 : Constant  Value=0
  Current Regulator (Ireg) : Subsystem
  DC Voltage Regulator (VDCreg) : Subsystem
  Demux1 : Demux  Outputs=2
  Demux3 : Demux  Outputs=2
  Detect Change : simulink/Logic and Bit Operations/Detect Change  Commented=on  vinit=0  OutDataTypeStr=boolean
  From13 : From  Commented=on  GotoTag=Pref  TagVisibility=global
  From20 : From  Commented=on  GotoTag=Qref  TagVisibility=global
  From25 : From  Commented=on  GotoTag=Brk2_On  TagVisibility=global
  From27 : From  Commented=on  GotoTag=Brk1_On  TagVisibility=global
  From37 : From  Commented=on  GotoTag=PQreg_On  TagVisibility=global
  From38 : From  Commented=on  GotoTag=VDCreg_On  TagVisibility=global
  Gain : Gain  Gain=1e-3
  Gain1 : Gain  Gain=-1
  Ground : Ground
  Ground1 : Ground
  Ground2 : Ground
  Mean : spsMeanLib/Mean  Freq=ConvCtrl.Freq/3  Vinit=0  Ts=ConvCtrl.Ts
  Mode of Operation Panel : Subsystem  Commented=on
  Mux : Mux  Inputs=2
  Mux1 : Mux  Inputs=2
  Mux2 : Mux  Inputs=2
  "PLL, Measurements and Transformation" : Subsystem
  Rate Transition{,1..3,7} (5 alike) : RateTransition  OutPortSampleTime=ConvCtrl.Ts
  Rate Transition11 : RateTransition  OutPortSampleTime=PlantSim.Ts
  Rate Transition6 : RateTransition  Commented=on  OutPortSampleTime=ConvCtrl.Ts
  Rate Transition8 : RateTransition  Commented=on  OutPortSampleTime=ConvCtrl.Ts
  Reactive Power Regulator : Subsystem
  Saturation Dynamic : simulink/Discontinuities/Saturation Dynamic  OutMin=[]  OutMax=[]  OutDataTypeStr=Inherit: Same as second input  OutDataType=fixdt(1, 16)  OutScaling=2^-10  DoSatur=off
  Scope2 : Scope  NumInputPorts=2
  Square : Math  Operator=square
  Square1 : Math  Operator=square
  Switch : Switch  Criteria=u2 ~= 0  SaturateOnIntegerOverflow=off  InputSameDT=off
  Uref : Outport
  Pmeas : Outport  Port=2
  Qmeas : Outport  Port=3
  fmeas : Outport  Port=4
  tag scope: IdMeas=global, IdRef=global, IqMeas=global, IqRef=global, delVd=global, delVq=global, meas1=global
  wires:
  Reactive Power Regulator/1(Qref_rpc) -> Mux2/1
  [Umeas] -> Reactive Power Regulator/2(Umeas)
  "PLL, Measurements and Transformation"/7(U_meas) -> [Umeas]  "Umeas"
  Rate Transition3/1 -> "PLL, Measurements and Transformation"/3(VPcc)
  VPcc/1 -> Rate Transition3/1
  [Vdc_meas] -> DC Voltage Regulator (VDCreg)/1(Vdc_meas), Scope2/1
  Rate Transition11/1 -> Uref/1  "Uref"
  From27/1 -> Rate Transition6/1
  Rate Transition8/1 -> Add1/2
  From25/1 -> Rate Transition8/1
  From37/1 -> Add1/4
  From38/1 -> Add1/3
  Rate Transition6/1 -> Add1/1
  Add1/1 -> Detect Change/1, Mode of Operation Panel/1(In1)
  Detect Change/1 -> Mode of Operation Panel/Enable
  [Pmeas] -> Mux1/2, Active Power Regulator (Preg)/1(Pmeas)
  "PLL, Measurements and Transformation"/6(Q) -> [Qmeas]
  [PrefPmeas] -> Bus Creator/7  "PrefPmeas"
  PrefPU/1 -> Mux1/1, Active Power Regulator (Preg)/2(Pref)
  Switch/1 -> DC Voltage Regulator (VDCreg)/2(Vdc_ref), Scope2/2
  [PQreg_On] -> Switch/2
  [Qmeas] -> Reactive Power Regulator/3(Qmes), Mux2/2
  [VdVq] -> Reactive Power Regulator/1(VdVq_mes)
  "PLL, Measurements and Transformation"/5(P) -> [Pmeas]
  Reactive Power Regulator/2(Iq_ref) -> [Iq_ref]
  Active Power Regulator (Preg)/1(Vdc_ref) -> [Vdc_ref_Preg]
  [PQreg_On] -> Active Power Regulator (Preg)/3(On)
  [VDCreg_On] -> DC Voltage Regulator (VDCreg)/3(On)
  [QrefQmeas] -> Bus Creator/8  "QrefQmeas"
  QrefPU/1 -> Reactive Power Regulator/4(Qref)
  [Vdc_ref_Preg] -> Switch/1
  Mux1/1 -> [PrefPmeas]
  Mux2/1 -> [QrefQmeas]
  [PQreg_On] -> Reactive Power Regulator/5(On)
  [Vdc_ref] -> Switch/3
  Rate Transition1/1 -> "PLL, Measurements and Transformation"/1(Vabc)
  Rate Transition7/1 -> Bus Creator/5  "m"
  Rate Transition2/1 -> "PLL, Measurements and Transformation"/2(Iabc)
  Rate Transition/1 -> [Vdc_meas], Gain/1
  [Iq_ref] -> Mux/2
  [VdVq] -> Current Regulator (Ireg)/3(VdVq)
  "PLL, Measurements and Transformation"/1(Freq) -> [Freq]  "Freq"
  [PIdq] -> Bus Creator/6  "PIdq"
  Demux1/1 -> Bus Creator/3  "Id"
  [m] -> Rate Transition7/1
  Demux3/2 -> Bus Creator/2  "Iqref"
  Bus Creator/1 -> [meas1]  "IBR_Control"
  [IdIq] -> Demux1/1
  Demux3/1 -> Bus Creator/1  "Idref"
  [IdIqref] -> Demux3/1
  [IdIq] -> Current Regulator (Ireg)/2(IdIq)
  Demux1/2 -> Bus Creator/4  "Iq"
  Mux/1 -> [IdIqref], Current Regulator (Ireg)/1(IdIq_ref)  "IdqRef"
  "PLL, Measurements and Transformation"/3(VdVq) -> [VdVq]  "VdqMeas"
  [Id_ref] -> Mux/1
  [Freq] -> Current Regulator (Ireg)/4(Freq)
  "PLL, Measurements and Transformation"/4(IdIq) -> [IdIq]  "IdqMeas"
  "PLL, Measurements and Transformation"/2(wt) -> [wt]  "wt"
  Vdc/1 -> Rate Transition/1
  [wt] -> Current Regulator (Ireg)/5(wt)
  Current Regulator (Ireg)/1(Uref_ABC) -> [Uref_ABC]
  Gain/1 -> Mean/1
  DC Voltage Regulator (VDCreg)/1(Id_ref) -> Saturation Dynamic/2
  [Vdc_meas] -> Current Regulator (Ireg)/6(Vdc)
  Isec/1 -> Rate Transition2/1
  Vsec/1 -> Rate Transition1/1
  Mean/1 -> [Vdc_kV]
  [Uref_ABC] -> Rate Transition11/1
  Constant/1 -> Square/1
  [Iq_ref] -> Square1/1
  Square/1 -> Add/1
  Square1/1 -> Add/2
  Add/1 -> Saturation Dynamic/1, Gain1/1
  Gain1/1 -> Saturation Dynamic/3
  Saturation Dynamic/1 -> [Id_ref]
  Ground/1 -> Pmeas/1
  Ground1/1 -> Qmeas/1
  Ground2/1 -> fmeas/1
  Bus Selector2/3 -> [IdMeas]  "<Id>"
  [meas1] -> Bus Selector2/1
  Bus Selector2/4 -> [IqMeas]  "<Iq>"
  Bus Selector2/2 -> [IqRef]  "<Iqref>"
  Bus Selector2/1 -> [IdRef]  "<Idref>"
  Constant1/1 -> [delVd]
  Constant2/1 -> [delVq]

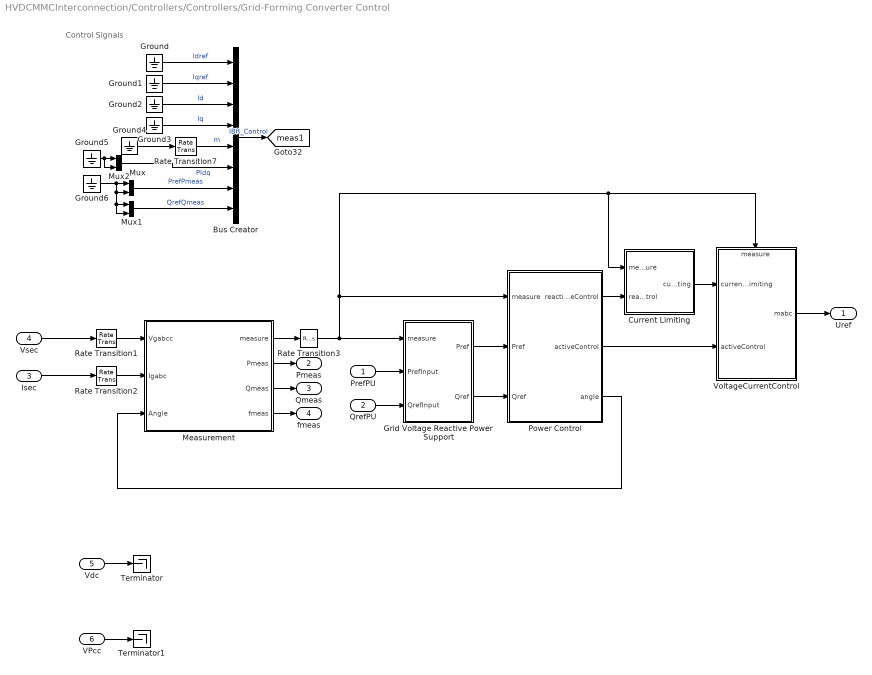
== system HVDCMMCInterconnection/Controllers/Controllers/Grid-Forming Converter Control ==
  note: Control Signals
  PrefPU : Inport
  QrefPU : Inport  Port=2
  Isec : Inport  Port=3
  Vsec : Inport  Port=4
  Vdc : Inport  Port=5
  VPcc : Inport  Port=6
  Bus Creator : BusCreator  Inputs=8
  Current Limiting : Subsystem
  Grid Voltage Reactive Power Support : Subsystem
  Ground{,1..6} (7 alike) : Ground
  Measurement : Subsystem
      mask Display: image('$imagefile'); % Use "Edit Image" on toolstrip to change.
  Mux : Mux  Inputs=2
  Mux1 : Mux  Inputs=2
  Mux2 : Mux  Inputs=2
  Power Control : Subsystem
  Rate Transition{1..3,7} (4 alike) : RateTransition  OutPortSampleTime=ConvCtrl.Ts
  Terminator : Terminator
  Terminator1 : Terminator
  VoltageCurrentControl : Subsystem
      settings: PortSchema="{\"entries\":[{\"content\":{\"sides\":[{\"content\":{\"connectorIds\":[\"In1\",\"In2\"]},\"type\":\"ConnectorPlacement.EquallySpacedRectSide\",\"uuid\":\"0bf15a12-7bc0-47e4-89bd-435769673763\"},{\"content\":{\"connectorIds\":[\"Out1\"],\"side\":\"RIGHT\"},\"type\":\"ConnectorPlacement.EquallySpacedRectSide\",\"uuid\":\"44a15d74-8878-4ec6-abe4-be0b1b609519\"},{\"content\":{\"connectorIds\":[\"In3\"],\"side\":\"TOP\"},\"type\":\"ConnectorPlacement.EquallySpacedRectSide\",\"uuid\":\"7a96781e-5638-4b2a-8101-d5785aae9f0f\"}]},\"type\":\"ConnectorPlacement.EquallySpacedConnector\",\"uuid\":\"4b3373ad-cf20-4175-894e-3bd1604dd0ce\"}],\"packageUris\":[\"http://schema.mathworks.com/mf0/Connector/R2020b\"],\"version\":\"1.0\"}"
  Uref : Outport
  Pmeas : Outport  Port=2
  Qmeas : Outport  Port=3
  fmeas : Outport  Port=4
  tag scope: meas1=global
  wires:
  VoltageCurrentControl/1(mabc) -> Uref/1
  Vsec/1 -> Rate Transition1/1
  Isec/1 -> Rate Transition2/1
  Measurement/2(Pmeas) -> Pmeas/1
  Measurement/3(Qmeas) -> Qmeas/1
  Measurement/1(measure) -> Rate Transition3/1
  Power Control/3(angle) -> Measurement/3(Angle)
  Power Control/1(reactiveControl) -> Current Limiting/2(reactiveControl)
  Current Limiting/1(currentLimiting) -> VoltageCurrentControl/1(currentLimiting)
  QrefPU/1 -> Grid Voltage Reactive Power Support/3(QrefInput)
  PrefPU/1 -> Grid Voltage Reactive Power Support/2(PrefInput)
  Grid Voltage Reactive Power Support/1(Pref) -> Power Control/2(Pref)
  Grid Voltage Reactive Power Support/2(Qref) -> Power Control/3(Qref)
  Measurement/4(fmeas) -> fmeas/1
  Rate Transition3/1 -> Current Limiting/1(measure), VoltageCurrentControl/3(measure), Power Control/1(measure), Grid Voltage Reactive Power Support/1(measure)
  Power Control/2(activeControl) -> VoltageCurrentControl/2(activeControl)
  Vdc/1 -> Terminator/1
  VPcc/1 -> Terminator1/1
  Ground2/1 -> Bus Creator/3  "Id"
  Bus Creator/1 -> [meas1]  "IBR_Control"
  Mux2/1 -> Bus Creator/6  "PIdq"
  Mux/1 -> Bus Creator/7  "PrefPmeas"
  Mux1/1 -> Bus Creator/8  "QrefQmeas"
  Rate Transition7/1 -> Bus Creator/5  "m"
  Ground/1 -> Bus Creator/1  "Idref"
  Ground3/1 -> Bus Creator/4  "Iq"
  Ground1/1 -> Bus Creator/2  "Iqref"
  Ground4/1 -> Rate Transition7/1
  Ground6/1 -> Mux/2, Mux1/2, Mux1/1, Mux/1
  Ground5/1 -> Mux2/2, Mux2/1
  Rate Transition1/1 -> Measurement/1(Vgabcc)
  Rate Transition2/1 -> Measurement/2(Igabc)

== system HVDCMMCInterconnection/Controllers/PWM Generators & Calculation of number of inserted modules (Nin) and number of blocked module (Nbl)/PWM Gen1 ==
  Uref : Inport
  Add6 : Sum
  Clock1 : DigitalClock  SampleTime=Ts
  Data Type Conversion : DataTypeConversion  OutDataTypeStr=double  SaturateOnIntegerOverflow=off  RndMeth=Floor
  Fc1 : Constant  Value=Tc
  Fc2 : Constant  Value=Fc
  Logical Operator2 : Logic  Operator=NOT  AllPortsSameDT=off  OutDataTypeStr=boolean
  Lookup Table1 : Lookup  InputValues=[0 .5 1]  Table=[-1 1 -1]  LookUpMeth=Interpolation-Use End Values  SaturateOnIntegerOverflow=off
  Math Function1 : Math  Operator=rem  SignedPower=on
  Mux6 : Mux  Inputs=2
  Phase_rad1 : Constant  Value=Offset_Cr
  Product2 : Product  RndMeth=Zero
  Relational Operator1 : RelationalOperator  OutDataTypeStr=boolean
  SelectPulses : Selector  InputPortWidth=2*n  IndexOptions=Index vector (dialog)  Indices=SelectPulsesPS  OutputSizes=1
  P : Outport
  Cr : Outport  Port=2
  wires:
  Data Type Conversion/1 -> P/1
  SelectPulses/1 -> Data Type Conversion/1
  Uref/1 -> Relational Operator1/1
  Lookup Table1/1 -> Relational Operator1/2, Cr/1
  Phase_rad1/1 -> Add6/2
  Fc2/1 -> Product2/2
  Logical Operator2/1 -> Mux6/2
  Mux6/1 -> SelectPulses/1
  Fc1/1 -> Math Function1/2
  Clock1/1 -> Add6/1
  Add6/1 -> Math Function1/1
  Product2/1 -> Lookup Table1/1
  Relational Operator1/1 -> Logical Operator2/1, Mux6/1
  Math Function1/1 -> Product2/1

== system HVDCMMCInterconnection/Controllers/PWM Generators & Calculation of number of inserted modules (Nin) and number of blocked module (Nbl)/PWM Gen2 ==
  Uref : Inport
  Add6 : Sum
  Clock1 : DigitalClock  SampleTime=Ts
  Data Type Conversion : DataTypeConversion  OutDataTypeStr=double  SaturateOnIntegerOverflow=off  RndMeth=Floor
  Fc1 : Constant  Value=Tc
  Fc2 : Constant  Value=Fc
  Logical Operator2 : Logic  Operator=NOT  AllPortsSameDT=off  OutDataTypeStr=boolean
  Lookup Table1 : Lookup  InputValues=[0 .5 1]  Table=[-1 1 -1]  LookUpMeth=Interpolation-Use End Values  SaturateOnIntegerOverflow=off
  Math Function1 : Math  Operator=rem  SignedPower=on
  Mux6 : Mux  Inputs=2
  Phase_rad1 : Constant  Value=Offset_Cr
  Product2 : Product  RndMeth=Zero
  Relational Operator1 : RelationalOperator  OutDataTypeStr=boolean
  SelectPulses : Selector  InputPortWidth=2*n  IndexOptions=Index vector (dialog)  Indices=SelectPulsesPS  OutputSizes=1
  P : Outport
  Cr : Outport  Port=2
  wires:
  Math Function1/1 -> Product2/1
  Relational Operator1/1 -> Mux6/1, Logical Operator2/1
  Product2/1 -> Lookup Table1/1
  Add6/1 -> Math Function1/1
  Clock1/1 -> Add6/1
  Fc1/1 -> Math Function1/2
  Mux6/1 -> SelectPulses/1
  Logical Operator2/1 -> Mux6/2
  Fc2/1 -> Product2/2
  Phase_rad1/1 -> Add6/2
  Lookup Table1/1 -> Cr/1, Relational Operator1/2
  Uref/1 -> Relational Operator1/1
  SelectPulses/1 -> Data Type Conversion/1
  Data Type Conversion/1 -> P/1

== system HVDCMMCInterconnection/Controllers/PWM Generators & Calculation of number of inserted modules (Nin) and number of blocked module (Nbl)/PWM Gen3 ==
  Uref : Inport
  Add6 : Sum
  Clock1 : DigitalClock  SampleTime=Ts
  Data Type Conversion : DataTypeConversion  OutDataTypeStr=double  SaturateOnIntegerOverflow=off  RndMeth=Floor
  Fc1 : Constant  Value=Tc
  Fc2 : Constant  Value=Fc
  Logical Operator2 : Logic  Operator=NOT  AllPortsSameDT=off  OutDataTypeStr=boolean
  Lookup Table1 : Lookup  InputValues=[0 .5 1]  Table=[-1 1 -1]  LookUpMeth=Interpolation-Use End Values  SaturateOnIntegerOverflow=off
  Math Function1 : Math  Operator=rem  SignedPower=on
  Mux6 : Mux  Inputs=2
  Phase_rad1 : Constant  Value=Offset_Cr
  Product2 : Product  RndMeth=Zero
  Relational Operator1 : RelationalOperator  OutDataTypeStr=boolean
  SelectPulses : Selector  InputPortWidth=2*n  IndexOptions=Index vector (dialog)  Indices=SelectPulsesPS  OutputSizes=1
  P : Outport
  Cr : Outport  Port=2
  wires:
  Data Type Conversion/1 -> P/1
  SelectPulses/1 -> Data Type Conversion/1
  Uref/1 -> Relational Operator1/1
  Lookup Table1/1 -> Relational Operator1/2, Cr/1
  Phase_rad1/1 -> Add6/2
  Fc2/1 -> Product2/2
  Logical Operator2/1 -> Mux6/2
  Mux6/1 -> SelectPulses/1
  Fc1/1 -> Math Function1/2
  Clock1/1 -> Add6/1
  Add6/1 -> Math Function1/1
  Product2/1 -> Lookup Table1/1
  Relational Operator1/1 -> Logical Operator2/1, Mux6/1
  Math Function1/1 -> Product2/1

== system HVDCMMCInterconnection/Controllers/PWM Generators & Calculation of number of inserted modules (Nin) and number of blocked module (Nbl)/PWM Gen4 ==
  Uref : Inport
  Add6 : Sum
  Clock1 : DigitalClock  SampleTime=Ts
  Data Type Conversion : DataTypeConversion  OutDataTypeStr=double  SaturateOnIntegerOverflow=off  RndMeth=Floor
  Fc1 : Constant  Value=Tc
  Fc2 : Constant  Value=Fc
  Logical Operator2 : Logic  Operator=NOT  AllPortsSameDT=off  OutDataTypeStr=boolean
  Lookup Table1 : Lookup  InputValues=[0 .5 1]  Table=[-1 1 -1]  LookUpMeth=Interpolation-Use End Values  SaturateOnIntegerOverflow=off
  Math Function1 : Math  Operator=rem  SignedPower=on
  Mux6 : Mux  Inputs=2
  Phase_rad1 : Constant  Value=Offset_Cr
  Product2 : Product  RndMeth=Zero
  Relational Operator1 : RelationalOperator  OutDataTypeStr=boolean
  SelectPulses : Selector  InputPortWidth=2*n  IndexOptions=Index vector (dialog)  Indices=SelectPulsesPS  OutputSizes=1
  P : Outport
  Cr : Outport  Port=2
  wires:
  Math Function1/1 -> Product2/1
  Relational Operator1/1 -> Mux6/1, Logical Operator2/1
  Product2/1 -> Lookup Table1/1
  Add6/1 -> Math Function1/1
  Clock1/1 -> Add6/1
  Fc1/1 -> Math Function1/2
  Mux6/1 -> SelectPulses/1
  Logical Operator2/1 -> Mux6/2
  Fc2/1 -> Product2/2
  Phase_rad1/1 -> Add6/2
  Lookup Table1/1 -> Cr/1, Relational Operator1/2
  Uref/1 -> Relational Operator1/1
  SelectPulses/1 -> Data Type Conversion/1
  Data Type Conversion/1 -> P/1

== system HVDCMMCInterconnection/Controllers/PWM Generators & Calculation of number of inserted modules (Nin) and number of blocked module (Nbl)/PWM Gen5 ==
  Uref : Inport
  Add6 : Sum
  Clock1 : DigitalClock  SampleTime=Ts
  Data Type Conversion : DataTypeConversion  OutDataTypeStr=double  SaturateOnIntegerOverflow=off  RndMeth=Floor
  Fc1 : Constant  Value=Tc
  Fc2 : Constant  Value=Fc
  Logical Operator2 : Logic  Operator=NOT  AllPortsSameDT=off  OutDataTypeStr=boolean
  Lookup Table1 : Lookup  InputValues=[0 .5 1]  Table=[-1 1 -1]  LookUpMeth=Interpolation-Use End Values  SaturateOnIntegerOverflow=off
  Math Function1 : Math  Operator=rem  SignedPower=on
  Mux6 : Mux  Inputs=2
  Phase_rad1 : Constant  Value=Offset_Cr
  Product2 : Product  RndMeth=Zero
  Relational Operator1 : RelationalOperator  OutDataTypeStr=boolean
  SelectPulses : Selector  InputPortWidth=2*n  IndexOptions=Index vector (dialog)  Indices=SelectPulsesPS  OutputSizes=1
  P : Outport
  Cr : Outport  Port=2
  wires:
  Data Type Conversion/1 -> P/1
  SelectPulses/1 -> Data Type Conversion/1
  Uref/1 -> Relational Operator1/1
  Lookup Table1/1 -> Relational Operator1/2, Cr/1
  Phase_rad1/1 -> Add6/2
  Fc2/1 -> Product2/2
  Logical Operator2/1 -> Mux6/2
  Mux6/1 -> SelectPulses/1
  Fc1/1 -> Math Function1/2
  Clock1/1 -> Add6/1
  Add6/1 -> Math Function1/1
  Product2/1 -> Lookup Table1/1
  Relational Operator1/1 -> Logical Operator2/1, Mux6/1
  Math Function1/1 -> Product2/1
